simulink model "simulink_control"  (R2024b)
settings: Solver=ode5  StartTime=0.0  StopTime=inf  FixedStep=0.064  RelTol=1e-3
values from neighbouring files (symbols this model uses):
  accelerometer_sensor = wb_robot_get_device('accelerometer')    [simulink_control_app.m]
  alpha_pitch = 0.85    [simulink_control_app.m]
  gps_sensor = wb_robot_get_device('gps')    [simulink_control_app.m]
  gyro_sensor = wb_robot_get_device('gyro')    [simulink_control_app.m]
  inertial_unit = wb_robot_get_device('inertial_unit')    [simulink_control_app.m]
  rotational_motor = wb_robot_get_device('rotational_motor')    [simulink_control_app.m]
  rotational_motor_propeller = wb_robot_get_device('rotational_motor_propeller')    [simulink_control_app.m]
  TIME_STEP = 16    [simulink_control_app.m]
libraries: robotalgslib x1
settings Model: Creator=Harun  LastModifiedBy=harunkurtdev

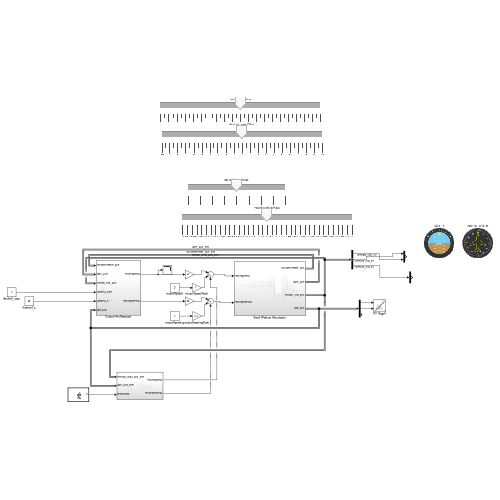
[thumbnail: Simulink's stored preview of the top-level diagram]
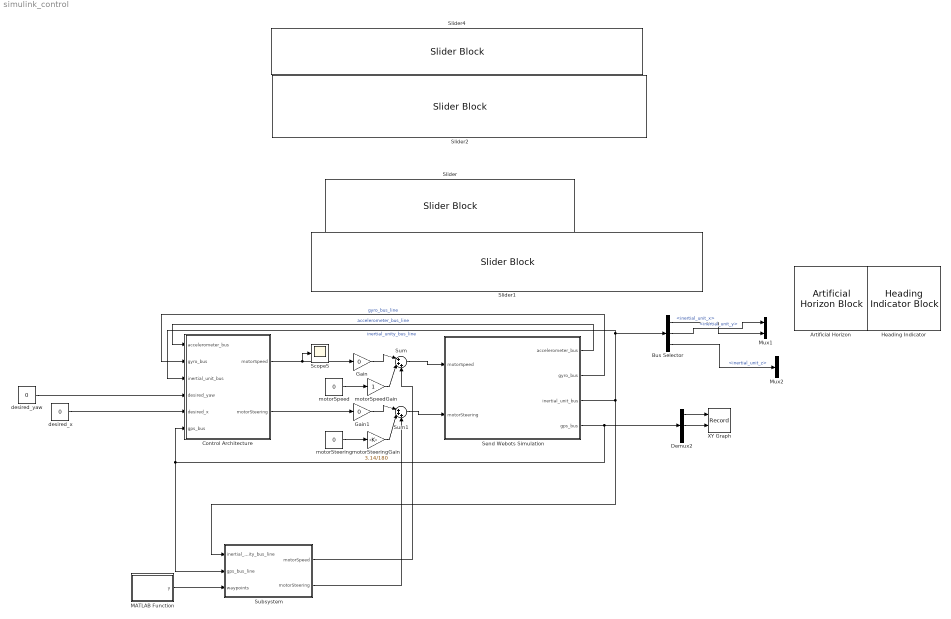
== system simulink_control ==
  Artificial Horizon : ArtificialHorizonBlock
  Bus Selector : BusSelector  OutputSignals=inertial_unit_x,inertial_unit_y,inertial_unit_z
  Control Architecture : Subsystem
  Demux2 : Demux  Outputs=3
  Gain : Gain  Gain=0
  Gain1 : Gain  Gain=0
  Heading Indicator : HeadingIndicatorBlock
  MATLAB Function : MATLAB Function  TreatAsAtomicUnit=on
  Mux1 : Mux  Inputs=2
  Mux2 : Mux  Inputs=1
  Scope5 : Scope
  Send Webots Simulation : Subsystem
  Slider : SliderBlock  ScaleMin=-10  ScaleMax=10  TickInterval=2.5
  Slider1 : SliderBlock  ScaleMin=-45  ScaleMax=45  TickInterval=2.5
  Slider2 : SliderBlock  ScaleMin=-10  ScaleMax=10  TickInterval=1
  Slider4 : SliderBlock  ScaleMin=-10  ScaleMax=10
  Subsystem : Subsystem
  Sum : Sum  Inputs=|+++
  Sum1 : Sum  Inputs=|+++
  XY Graph : Record  FileSettingsInternal="{\"entries\":[{\"content\":{\"excelSettings\":{\"content\":{},\"type\":\"Streamout.ExcelSettings\"}},\"type\":\"Streamout.FileSettingStorage\",\"uuid\":\"\"}],\"packageUris\":[\"http:\\/\\/schema.mathworks.com\\/mf0\\/streamout_blocks\\/R2020a\"],\"version\":\"1.0\"}"  Layout=[1 1]  SignalsInternal="{\"entries\":[{\"content\":{\"signals\":[{\"content\":{\"blockPath\":[],\"dimensions\":[1],\"domain\":\"\",\"lineColor\":\"#a2142f\",\"plots\":[ 1 ],\"port\":1,\"sid\":[\"\"],\"signalID\":1,\"signalName\":\"Demux2:1\"},\"type\":\"RecordBlkView.Signal\",\"uuid\":\"\"},{\"content\":{\"blockPath\":[],\"dimensions\":[1],\"domain\":\"\",\"lineColor\":\"#139fff\",\"plots\":[ 1 ],\"port\":2,\"sid\":[\"\"],\"signalID\":2,\"signalName\":\"Demux2:2\"},\"type\":\"RecordBlkView.Signal\",\"uuid\":\"\"}]},\"type\":\"RecordBlkView.InputSignals\",\"uuid\":\"\"}],\"packageUris\":[\"http:\\/\\/schema.mathworks.com\\/mf0\\/streamout_blocks\\/R2020a\"],\"version\":\"1.0\"}"  VisualizationBindings="{\"xyplotplugin\":{\"info\":[{\"series\":[{\"bindingParametersList\":[{\"parameter\":\"X-Axis\",\"signalID\":1,\"signalName\":\"Demux2:1\"},{\"parameter\":\"Y-Axis\",\"signalID\":2,\"signalName\":\"Demux2:2\"}],\"seriesID\":0}],\"subplotID\":1}]}}"  CompatibilityTag=XY
  desired_x : Constant  Value=0
  desired_yaw : Constant  Value=0
  motorSpeed : Constant  Value=0
  motorSpeedGain : Gain
  motorSteering : Constant  Value=0
  motorSteeringGain : Gain  Gain=3.14/180
  wires:
  motorSteering/1 -> motorSteeringGain/1
  motorSpeed/1 -> motorSpeedGain/1
  Sum/1 -> Send Webots Simulation/1(motorSpeed)
  Control Architecture/1(motorSpeed) -> Scope5/1, Gain/1
  Control Architecture/2(motorSteering) -> Gain1/1
  Sum1/1 -> Send Webots Simulation/2(motorSteering)
  motorSpeedGain/1 -> Sum/2
  motorSteeringGain/1 -> Sum1/2
  desired_yaw/1 -> Control Architecture/4(desired_yaw)
  Send Webots Simulation/1(accelerometer_bus) -> Control Architecture/1(accelerometer_bus)  "accelerometer_bus_line"
  Send Webots Simulation/2(gyro_bus) -> Control Architecture/2(gyro_bus)  "gyro_bus_line"
  Send Webots Simulation/3(inertial_unit_bus) -> Subsystem/1(inertial_unity_bus_line), Control Architecture/3(inertial_unit_bus), Bus Selector/1  "inertial_unity_bus_line"
  Gain/1 -> Sum/1
  Gain1/1 -> Sum1/1
  desired_x/1 -> Control Architecture/5(desired_x)
  Send Webots Simulation/4(gps_bus) -> Subsystem/2(gps_bus_line), Control Architecture/6(gps_bus), Demux2/1
  Demux2/1 -> XY Graph/1
  Demux2/2 -> XY Graph/2
  Bus Selector/1 -> Mux1/2  "<inertial_unit_x>"
  Bus Selector/2 -> Mux1/1  "<inertial_unit_y>"
  Bus Selector/3 -> Mux2/1  "<inertial_unit_z>"
  MATLAB Function/1(y) -> Subsystem/3(waypoints)
  Subsystem/1(motorSpeed) -> Sum/3
  Subsystem/2(motorSteering) -> Sum1/3

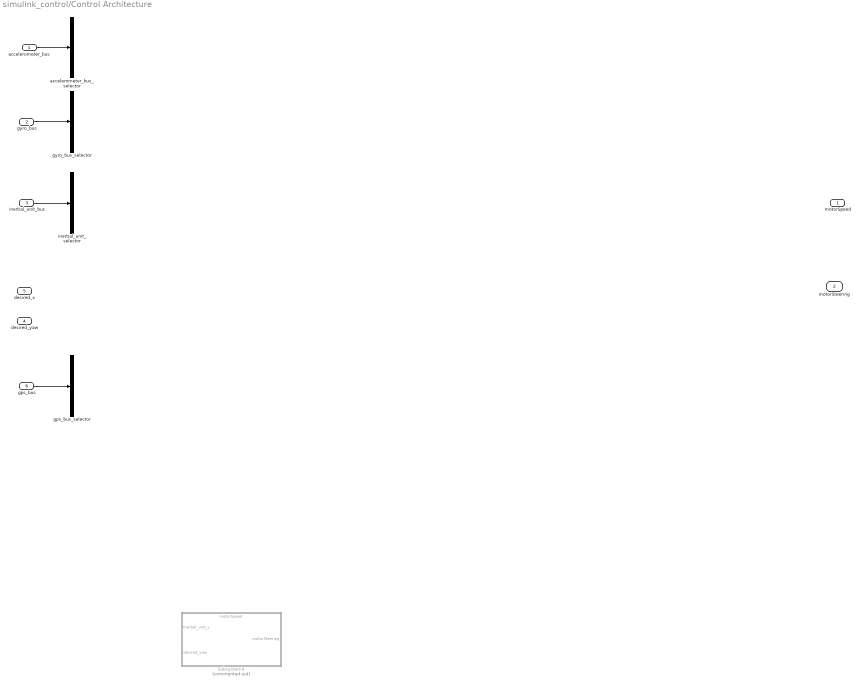
== system simulink_control/Control Architecture ==
  accelerometer_bus : Inport
  gyro_bus : Inport  Port=2
  inertial_unit_bus : Inport  Port=3
  desired_yaw : Inport  Port=4
  desired_x : Inport  Port=5
  gps_bus : Inport  Port=6
  Subsystem4 : Subsystem  Commented=on
      settings: PortSchema="{\"entries\":[{\"content\":{\"sides\":[{\"content\":{\"connectorIds\":[\"In1\",\"In2\"]},\"type\":\"ConnectorPlacement.EquallySpacedRectSide\",\"uuid\":\"8ea77c90-69e3-4b28-847a-36c3733c4ca1\"},{\"content\":{\"connectorIds\":[\"Out1\"],\"side\":\"RIGHT\"},\"type\":\"ConnectorPlacement.EquallySpacedRectSide\",\"uuid\":\"94f1f4b2-c797-44bf-abc2-6d3fe195cf34\"},{\"content\":{\"connectorIds\":[\"In3\"],\"side\":\"TOP\"},\"type\":\"ConnectorPlacement.EquallySpacedRectSide\",\"uuid\":\"06572095-9567-46cb-bcf7-b6a4abacf0e1\"}]},\"type\":\"ConnectorPlacement.EquallySpacedConnector\",\"uuid\":\"9f096835-0cc4-4d1f-8b4a-1f4eeb97a32d\"}],\"packageUris\":[\"http://schema.mathworks.com/mf0/Connector/R2020b\"],\"version\":\"1.0\"}"
  accelerometer_bus_selector : BusSelector  OutputSignals=accelerometer_x,accelerometer_y,accelerometer_z
  gps_bus_selector : BusSelector  OutputSignals=gps_x,gps_y,gps_z
  gyro_bus_selector : BusSelector  OutputSignals=gyro_x,gyro_y,gyro_z
  inertial_unit_selector : BusSelector  OutputSignals=inertial_unit_x,inertial_unit_y,inertial_unit_z
  motorSpeed : Outport
  motorSteering : Outport  Port=2
  wires:
  accelerometer_bus/1 -> accelerometer_bus_selector/1
  gyro_bus/1 -> gyro_bus_selector/1
  inertial_unit_bus/1 -> inertial_unit_selector/1
  gps_bus/1 -> gps_bus_selector/1

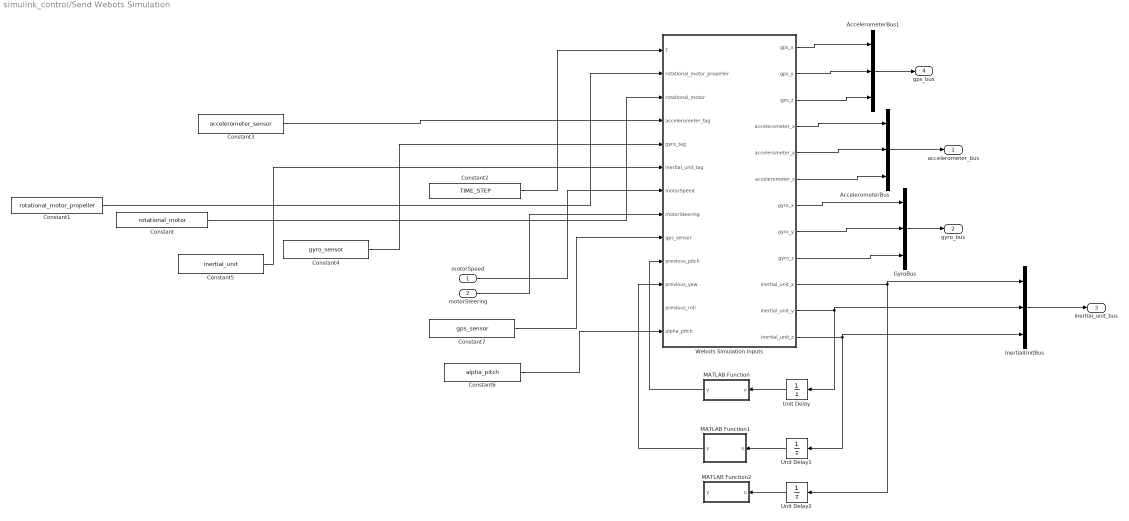
== system simulink_control/Send Webots Simulation ==
  motorSpeed : Inport
  motorSteering : Inport  Port=2
  AccelerometerBus : BusCreator  Inputs=3
  AccelerometerBus1 : BusCreator  Inputs=3
  Constant : Constant  Value=rotational_motor
  Constant1 : Constant  Value=rotational_motor_propeller
  Constant2 : Constant  Value=TIME_STEP
  Constant3 : Constant  Value=accelerometer_sensor
  Constant4 : Constant  Value=gyro_sensor
  Constant5 : Constant  Value=inertial_unit
  Constant6 : Constant  Value=alpha_pitch
  Constant7 : Constant  Value=gps_sensor
  GyroBus : BusCreator  Inputs=3
  InertialUnitBus : BusCreator  Inputs=3
  MATLAB Function : MATLAB Function  TreatAsAtomicUnit=on
  MATLAB Function1 : MATLAB Function  TreatAsAtomicUnit=on
  MATLAB Function2 : MATLAB Function  TreatAsAtomicUnit=on
  Unit Delay : UnitDelay  SampleTime=-1  HasFrameUpgradeWarning=on
  Unit Delay1 : UnitDelay  SampleTime=-1  HasFrameUpgradeWarning=on
  Unit Delay2 : UnitDelay  SampleTime=-1  HasFrameUpgradeWarning=on
  Webots Simulation Inputs : MATLAB Function  TreatAsAtomicUnit=on
  accelerometer_bus : Outport
  gyro_bus : Outport  Port=2
  inertial_unit_bus : Outport  Port=3
  gps_bus : Outport  Port=4
  wires:
  motorSpeed/1 -> Webots Simulation Inputs/7(motorSpeed)
  Constant/1 -> Webots Simulation Inputs/3(rotational_motor)
  Constant2/1 -> Webots Simulation Inputs/1(T)
  Constant1/1 -> Webots Simulation Inputs/2(rotational_motor_propeller)
  Webots Simulation Inputs/5(accelerometer_y) -> AccelerometerBus/2
  Webots Simulation Inputs/4(accelerometer_x) -> AccelerometerBus/1
  Webots Simulation Inputs/6(accelerometer_z) -> AccelerometerBus/3
  AccelerometerBus/1 -> accelerometer_bus/1
  Constant3/1 -> Webots Simulation Inputs/4(accelerometer_tag)
  motorSteering/1 -> Webots Simulation Inputs/8(motorSteering)
  Constant4/1 -> Webots Simulation Inputs/5(gyro_tag)
  Webots Simulation Inputs/9(gyro_z) -> GyroBus/3
  Webots Simulation Inputs/8(gyro_y) -> GyroBus/2
  GyroBus/1 -> gyro_bus/1
  Webots Simulation Inputs/7(gyro_x) -> GyroBus/1
  Webots Simulation Inputs/10(inertial_unit_x) -> InertialUnitBus/1, Unit Delay2/1
  Webots Simulation Inputs/11(inertial_unit_y) -> InertialUnitBus/2, Unit Delay/1
  Webots Simulation Inputs/12(inertial_unit_z) -> InertialUnitBus/3, Unit Delay1/1
  InertialUnitBus/1 -> inertial_unit_bus/1
  Constant5/1 -> Webots Simulation Inputs/6(inertial_unit_tag)
  Constant6/1 -> Webots Simulation Inputs/13(alpha_pitch)
  MATLAB Function/1(y) -> Webots Simulation Inputs/10(previous_pitch)
  Unit Delay/1 -> MATLAB Function/1(u)
  Unit Delay1/1 -> MATLAB Function1/1(u)
  MATLAB Function1/1(y) -> Webots Simulation Inputs/11(previous_yaw)
  Constant7/1 -> Webots Simulation Inputs/9(gps_sensor)
  Webots Simulation Inputs/1(gps_x) -> AccelerometerBus1/1
  Webots Simulation Inputs/2(gps_y) -> AccelerometerBus1/2
  Webots Simulation Inputs/3(gps_z) -> AccelerometerBus1/3
  AccelerometerBus1/1 -> gps_bus/1
  Unit Delay2/1 -> MATLAB Function2/1(u)

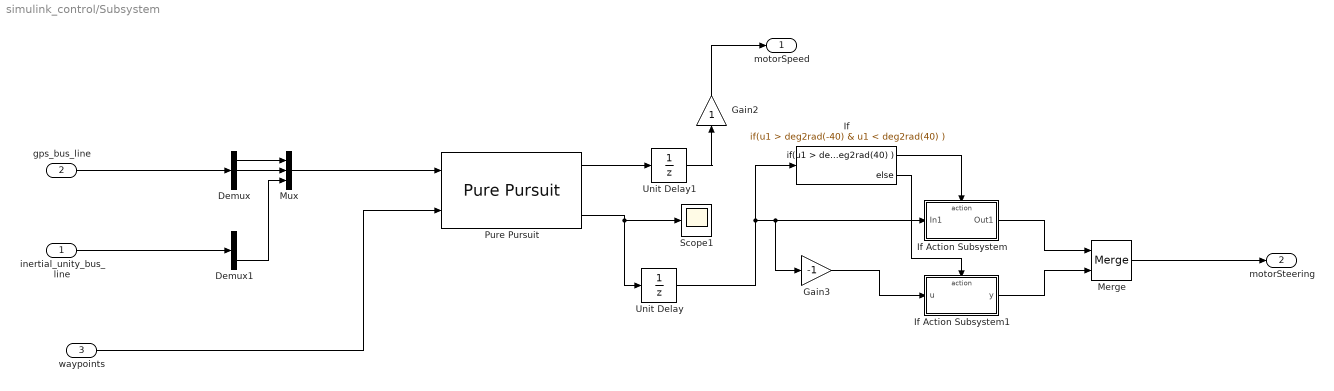
== system simulink_control/Subsystem ==
  inertial_unity_bus_line : Inport
  gps_bus_line : Inport  Port=2
  waypoints : Inport  Port=3
  Demux : Demux  Outputs=3
  Demux1 : Demux  Outputs=3
  Gain2 : Gain
  Gain3 : Gain  Gain=-1
  If : If  IfExpression=u1 > deg2rad(-40) & u1 < deg2rad(40)
  If Action Subsystem : Subsystem  TreatAsAtomicUnit=on
  If Action Subsystem1 : Subsystem  TreatAsAtomicUnit=on
  Merge : Merge
  Mux : Mux  Inputs=3
  Pure Pursuit : robotalgslib/Pure Pursuit  DesiredLinearVelocityPort=off  DesiredLinearVelocity=2.5  MaxAngularVelocity=1.0  LookaheadDistancePort=off  LookaheadDistance=1.0  TargetDirPort=on  SimulateUsing=Code generation
      settings: LibrarySourceBlock=navlib/Control Algorithms/Pure Pursuit
  Scope1 : Scope
  Unit Delay : UnitDelay  SampleTime=-1  HasFrameUpgradeWarning=on
  Unit Delay1 : UnitDelay  SampleTime=-1  HasFrameUpgradeWarning=on
  motorSpeed : Outport
  motorSteering : Outport  Port=2
  wires:
  If/2 -> If Action Subsystem1/Action
  Gain2/1 -> motorSpeed/1
  Pure Pursuit/3 -> Unit Delay/1, Scope1/1
  Demux/1 -> Mux/1
  Demux/2 -> Mux/2
  gps_bus_line/1 -> Demux/1
  Merge/1 -> motorSteering/1
  If Action Subsystem1/1(y) -> Merge/2
  If/1 -> If Action Subsystem/Action
  Gain3/1 -> If Action Subsystem1/1(u)
  inertial_unity_bus_line/1 -> Demux1/1
  Unit Delay1/1 -> Gain2/1
  Mux/1 -> Pure Pursuit/1
  If Action Subsystem/1(Out1) -> Merge/1
  waypoints/1 -> Pure Pursuit/2
  Unit Delay/1 -> If/1, Gain3/1, If Action Subsystem/1(In1)
  Pure Pursuit/1 -> Unit Delay1/1
  Demux1/3 -> Mux/3

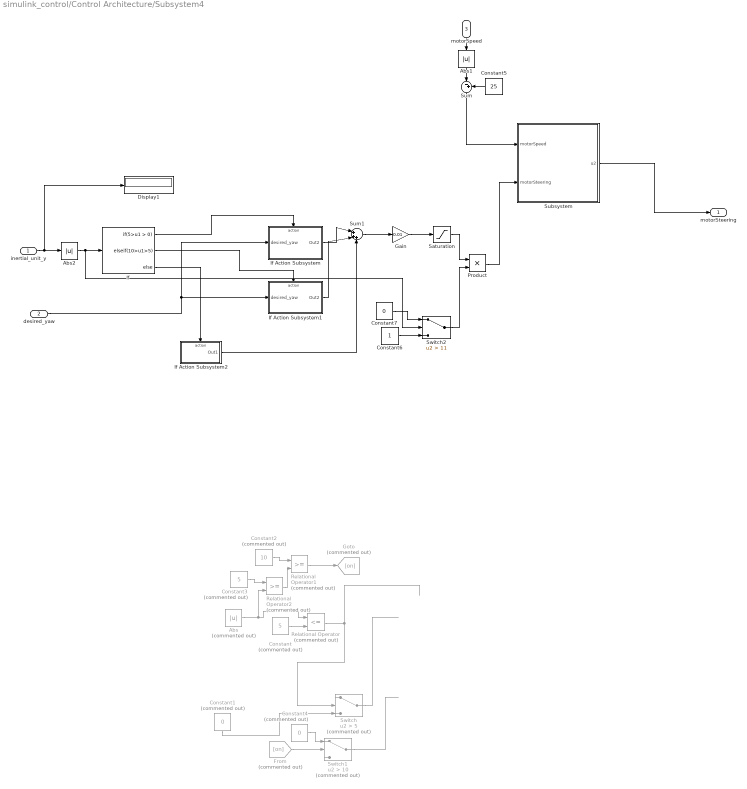
== system simulink_control/Control Architecture/Subsystem4 ==
  inertial_unit_y : Inport
  desired_yaw : Inport  Port=2
  motorSpeed : Inport  Port=3
  Abs : Abs  Commented=on  SaturateOnIntegerOverflow=off
  Abs1 : Abs  SaturateOnIntegerOverflow=off
  Abs2 : Abs  SaturateOnIntegerOverflow=off
  Constant : Constant  Commented=on  Value=5
  Constant1 : Constant  Commented=on  Value=0
  Constant2 : Constant  Commented=on  Value=10
  Constant3 : Constant  Commented=on  Value=5
  Constant4 : Constant  Commented=on  Value=0
  Constant5 : Constant  Value=25
  Constant6 : Constant
  Constant7 : Constant  Value=0
  Display1 : Display
  From : From  Commented=on  GotoTag=on
  Gain : Gain  Gain=0.01
  Goto : Goto  Commented=on  GotoTag=on
  If : If  IfExpression=5>u1 > 0  ElseIfExpressions=10>u1>5
  If Action Subsystem : Subsystem  TreatAsAtomicUnit=on
  If Action Subsystem1 : Subsystem  TreatAsAtomicUnit=on
  If Action Subsystem2 : Subsystem  TreatAsAtomicUnit=on
  Product : Product
  Relational Operator : RelationalOperator  Commented=on  Operator=<=  OutDataTypeStr=boolean  RndMeth=Simplest  InputSameDT=off
  Relational Operator1 : RelationalOperator  Commented=on  OutDataTypeStr=boolean  RndMeth=Simplest  InputSameDT=off
  Relational Operator2 : RelationalOperator  Commented=on  OutDataTypeStr=boolean  RndMeth=Simplest  InputSameDT=off
  Saturation : Saturate  UpperLimit=1000  LowerLimit=-1000
  Subsystem : Subsystem
  Sum : Sum  Inputs=|-+
  Sum1 : Sum  Inputs=|+++
  Switch : Switch  Commented=on  Criteria=u2 > Threshold  Threshold=5  SaturateOnIntegerOverflow=off  InputSameDT=off
  Switch1 : Switch  Commented=on  Criteria=u2 > Threshold  Threshold=10  SaturateOnIntegerOverflow=off  InputSameDT=off
  Switch2 : Switch  Criteria=u2 > Threshold  Threshold=11  SaturateOnIntegerOverflow=off  InputSameDT=off
  motorSteering : Outport
  wires:
  motorSpeed/1 -> Abs1/1
  Abs1/1 -> Sum/1
  Constant5/1 -> Sum/2
  Constant1/1 -> Switch/3
  From/1 -> Switch1/2
  Constant4/1 -> Switch1/1
  Switch1/1 -> ?
  Constant/1 -> Relational Operator/2
  Relational Operator1/1 -> Goto/1
  Constant3/1 -> Relational Operator2/1
  Abs/1 -> Relational Operator2/2, Relational Operator/1
  ? -> Switch1/3, Switch/1
  Constant2/1 -> Relational Operator1/1
  Switch/1 -> ?
  Relational Operator2/1 -> Relational Operator1/2
  Relational Operator/1 -> Switch/2
  inertial_unit_y/1 -> Display1/1, Abs2/1
  If/3 -> If Action Subsystem2/Action
  Abs2/1 -> Switch2/2, If/1
  If/1 -> If Action Subsystem/Action
  If Action Subsystem1/1(Out2) -> Sum1/2
  If Action Subsystem/1(Out2) -> Sum1/1
  If/2 -> If Action Subsystem1/Action
  Sum1/1 -> Gain/1
  Gain/1 -> Saturation/1
  Sum/1 -> Subsystem/1(motorSpeed)
  Saturation/1 -> Product/1
  Constant6/1 -> Switch2/3
  Constant7/1 -> Switch2/1
  Switch2/1 -> Product/2
  Product/1 -> Subsystem/2(motorSteering)
  If Action Subsystem2/1(Out1) -> Sum1/3
  desired_yaw/1 -> If Action Subsystem/1(desired_yaw), If Action Subsystem1/1(desired_yaw)
  Subsystem/1(u2) -> motorSteering/1

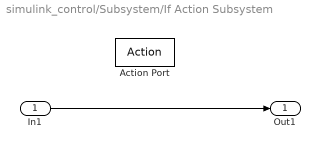
== system simulink_control/Subsystem/If Action Subsystem ==
  In1 : Inport
  Action Port : ActionPort  ActionPortLabel=|
      | if(u1 > deg2rad(-40) & u1 < deg2rad(40)
      | )
  Out1 : Outport
  wires:
  In1/1 -> Out1/1

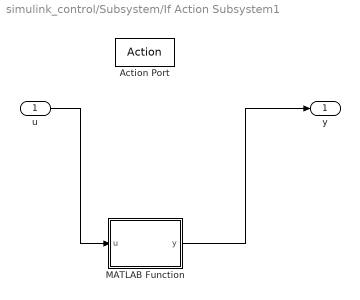
== system simulink_control/Subsystem/If Action Subsystem1 ==
  u : Inport
  Action Port : ActionPort  ActionPortLabel=else
  MATLAB Function : MATLAB Function  TreatAsAtomicUnit=on
  y : Outport
  wires:
  u/1 -> MATLAB Function/1(u)
  MATLAB Function/1(y) -> y/1

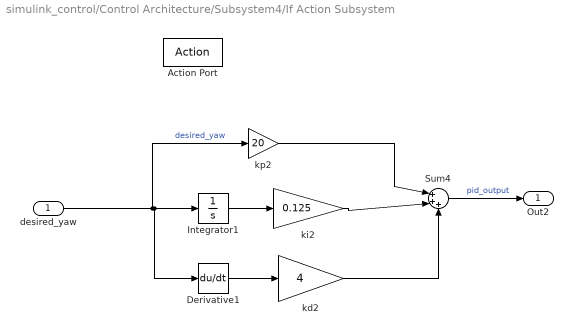
== system simulink_control/Control Architecture/Subsystem4/If Action Subsystem ==
  desired_yaw : Inport
  Action Port : ActionPort
  Derivative1 : Derivative  CoefficientInTFapproximation=0.016
  Integrator1 : Integrator
  Sum4 : Sum  Inputs=|+++
  kd2 : Gain  Gain=4
  ki2 : Gain  Gain=0.125
  kp2 : Gain  Gain=20
  Out2 : Outport
  wires:
  Derivative1/1 -> kd2/1
  Sum4/1 -> Out2/1  "pid_output"
  kp2/1 -> Sum4/1
  ki2/1 -> Sum4/2
  Integrator1/1 -> ki2/1
  desired_yaw/1 -> kp2/1, Derivative1/1, Integrator1/1  "desired_yaw"
  kd2/1 -> Sum4/3

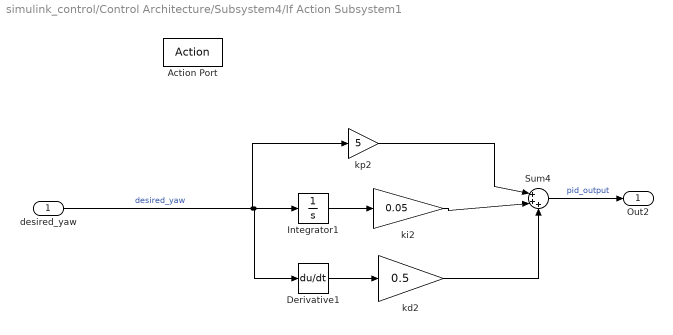
== system simulink_control/Control Architecture/Subsystem4/If Action Subsystem1 ==
  desired_yaw : Inport
  Action Port : ActionPort
  Derivative1 : Derivative  CoefficientInTFapproximation=0.016
  Integrator1 : Integrator
  Sum4 : Sum  Inputs=|+++
  kd2 : Gain  Gain=0.5
  ki2 : Gain  Gain=0.05
  kp2 : Gain  Gain=5
  Out2 : Outport
  wires:
  Derivative1/1 -> kd2/1
  Sum4/1 -> Out2/1  "pid_output"
  kp2/1 -> Sum4/1
  ki2/1 -> Sum4/2
  Integrator1/1 -> ki2/1
  desired_yaw/1 -> kp2/1, Derivative1/1, Integrator1/1  "desired_yaw"
  kd2/1 -> Sum4/3

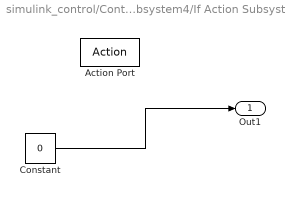
== system simulink_control/Control Architecture/Subsystem4/If Action Subsystem2 ==
  Action Port : ActionPort
  Constant : Constant  Value=0
  Out1 : Outport
  wires:
  Constant/1 -> Out1/1

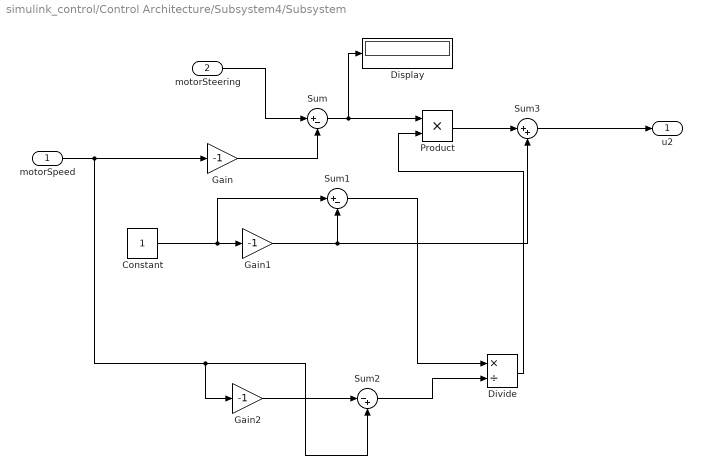
== system simulink_control/Control Architecture/Subsystem4/Subsystem ==
  motorSpeed : Inport
  motorSteering : Inport  Port=2
  Constant : Constant
  Display : Display
  Divide : Product  Inputs=*/
  Gain : Gain  Gain=-1
  Gain1 : Gain  Gain=-1
  Gain2 : Gain  Gain=-1
  Product : Product
  Sum : Sum  Inputs=|+-
  Sum1 : Sum  Inputs=|+-
  Sum2 : Sum  Inputs=|-+
  Sum3 : Sum  Inputs=|++
  u2 : Outport
  wires:
  Sum3/1 -> u2/1
  Product/1 -> Sum3/1
  Divide/1 -> Product/2
  Sum1/1 -> Divide/1
  Sum2/1 -> Divide/2
  Gain2/1 -> Sum2/1
  motorSpeed/1 -> Gain2/1, Sum2/2, Gain/1
  Constant/1 -> Gain1/1, Sum1/1
  Gain1/1 -> Sum1/2, Sum3/2
  Sum/1 -> Display/1, Product/1
  Gain/1 -> Sum/2
  motorSteering/1 -> Sum/1

== matlab function simulink_control/MATLAB Function ==
  data: y output
function y = fcn()

y = [0,0;2,3;0,5;10,10];

== matlab function simulink_control/Send Webots Simulation/Webots Simulation Inputs ==
  data: gps_x output; gps_y output; gps_z output; T input; rotational_motor_propeller input; rotational_motor input; accelerometer_tag input; gyro_tag input; inertial_unit_tag input; motorSpeed input; accelerometer_x output; accelerometer_y output; accelerometer_z output; motorSteering input; gps_sensor input; gyro_x output; gyro_y output; gyro_z output; inertial_unit_x output; inertial_unit_y output; inertial_unit_z output; previous_pitch input; previous_yaw input; previous_roll input; alpha_pitch input
function [gps_x,gps_y,gps_z,accelerometer_x,accelerometer_y,accelerometer_z,gyro_x,gyro_y,gyro_z,inertial_unit_x,inertial_unit_y,inertial_unit_z] = simulation(T,rotational_motor_propeller,rotational_motor,accelerometer_tag,gyro_tag,inertial_unit_tag ...
    ,motorSpeed,motorSteering,gps_sensor,previous_pitch,previous_yaw,previous_roll,alpha_pitch)


accelerometer_x = 0.0;
accelerometer_y = 0.0;
accelerometer_z = 0.0;

gyro_x=0.0;
gyro_y=0.0;
gyro_z=0.0;

gps_x=0.0;
gps_y=0.0;
gps_z=0.0;

wb_robot_step(T)
wb_motor_set_position(rotational_motor_propeller, Inf);
%wb_motor_set_position(rotational_motor, Inf);
wb_motor_set_position(rotational_motor, motorSteering);
wb_motor_set_velocity(rotational_motor_propeller, motorSpeed);

%period = wb_accelerometer_get_sampling_period(accelerometer_tag)
accelerometer_values = zeros(1, 3); 
accelerometer_values = wb_accelerometer_get_values(accelerometer_tag);
accelerometer_x = accelerometer_values(1);
accelerometer_y = accelerometer_values(2);
accelerometer_z = accelerometer_values(3);

gps_values= zeros(1,3);
gps_values=wb_gps_get_values(gps_sensor);

gps_x=gps_values(1);
gps_y=gps_values(2);
gps_z=gps_values(3);


gyro_values = zeros(1, 3); 
gyro_values = wb_gyro_get_values(gyro_tag);

gyro_x = gyro_values(1);
gyro_y = gyro_values(2);
gyro_z = gyro_values(3);


inertial_unit_values = zeros(1, 3); 
inertial_unit_values = wb_inertial_unit_get_roll_pitch_yaw(inertial_unit_tag);



inertial_unit_x = inertial_unit_values(1);
inertial_unit_y = inertial_unit_values(2);
inertial_unit_z = inertial_unit_values(3);

interial_unit_y=alpha_pitch*inertial_unit_y+(1-alpha_pitch)*previous_pitch;

inertial_unit_z=alpha_pitch*inertial_unit_z+(1-alpha_pitch)*previous_yaw;
interial_unit_x= alpha_pitch*inertial_unit_x+ (1-alpha_pitch)*previous_roll;



end

== matlab function simulink_control/Send Webots Simulation/MATLAB Function2 ==
  data: u input; y output
function y = fcn(u)

y = u;

== matlab function simulink_control/Subsystem/If Action Subsystem1/MATLAB Function ==
  data: u input; y output
function y = fcn(u)

y = zeros(1,1);
if (u<=deg2rad(-40)) || (u>=deg2rad(40))
    disp('u is outside ');
else 
    y = -u;

end

== matlab function simulink_control/Send Webots Simulation/MATLAB Function ==
  data: u input; y output
function y = fcn(u)

y = u;

== matlab function simulink_control/Send Webots Simulation/MATLAB Function1 ==
  data: u input; y output
function y = fcn(u)

y = u;
